simulink model "RL_Model_dyn"  (R2020a)
settings: Solver=FixedStepAuto  StartTime=0.0  StopTime=80  FixedStep=1E-3  MaxStep=0.01  MinStep=1e-3  RelTol=1e-3
model workspace (MAT data in the model file):
  reward_sys.DE_penalty_gain = 15
  reward_sys.DE_penalty_shape = 2
  reward_sys.HE_penalty_gain = 20
  reward_sys.HE_penalty_shape = 2
  reward_sys.HE_iwrt_DE = 1.5
  reward_sys.vel_reward_gain = 0
  reward_sys.vel_iwrt_DE = 1
  reward_sys.steering_penalty_gain = 0.1
  reward_sys.steering_iwrt_DE = 1
  reward_sys.steering_iwrt_HE = 1
values from neighbouring files (symbols this model uses):
  CP_Num = CP_Base_Num + CP_Wheels_Num    [init_Dmodel_sim_vars.m]
  D = 1000    [init_Dmodel_sim_vars.m]
  K = 1e6    (= 1000000)    [init_Dmodel_sim_vars.m]
  model = floatbase(model)    [init_Dmodel_sim_vars.m]
  Mu = 0.8    [init_Dmodel_sim_vars.m]
  q_init = [0 0 0 0]'    [init_Dmodel_sim_vars.m]
  qd_init = [0 0 0 0]'    [init_Dmodel_sim_vars.m]
  R = 0.1    [init_Dmodel_sim_vars.m]
  x_init = [1 0 0 0  0 0 zoff   0 0 0  2 0 0]'    [init_Dmodel_sim_vars.m]
undefined symbols (not defined in the file or in its folder): DiscIntNeverNeededParam, Fpt, gcontact, gcPosVel
libraries: simulink x7, rllib x1
settings Model: Creator=12248  LastModifiedBy=sky32
settings SolverCC: ZeroCrossAlgorithm=Adaptive
settings DataIOCC: SignalLogging=off
settings SFSimCC: CustomCodeUndefinedFunction=UseInterfaceOnly

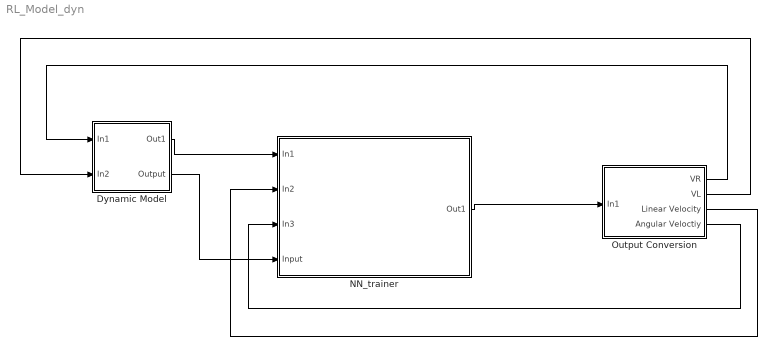
== system RL_Model_dyn ==
  Dynamic Model : Subsystem
  NN_trainer : Subsystem
  Output Conversion : Subsystem
  wires:
  NN_trainer/1(Out1) -> Output Conversion/1(In1)
  Dynamic Model/1(Out1) -> NN_trainer/1(In1)
  Output Conversion/4(Angular Veloctiy) -> NN_trainer/3(In3)
  Output Conversion/3(Linear Velocity) -> NN_trainer/2(In2)
  Output Conversion/1(VR) -> Dynamic Model/1(In1)
  Output Conversion/2(VL) -> Dynamic Model/2(In2)
  Dynamic Model/2(Output) -> NN_trainer/4(Input)

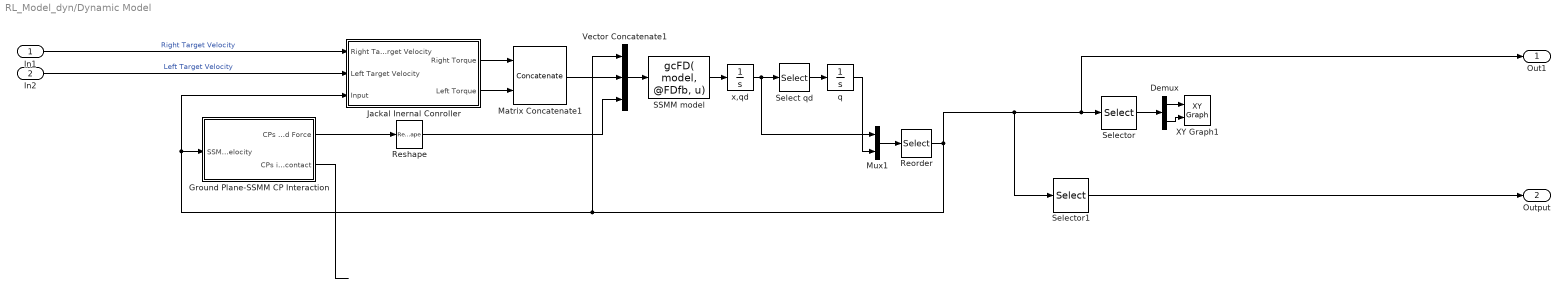
== system RL_Model_dyn/Dynamic Model ==
  In1 : Inport
  In2 : Inport  Port=2
  Demux : Demux  Outputs=2
  Ground Plane-SSMM CP Interaction : Subsystem
  Jackal Inernal Conroller : Subsystem
  Matrix Concatenate1 : Concatenate  Mode=Multidimensional array
  Mux1 : Mux  Inputs=2
  Reorder : Selector  InputPortWidth=21  IndexOptions=Index vector (dialog)  Indices=[1 2 3 4 5 6 7 8 9 10 11 12 13 18 19 20 21 14 15 16 17]  OutputSizes=1
  Reshape : Reshape  OutputDimensionality=Column vector (2-D)
  SSMM model : MATLABFcn  MATLABFcn=gcFD( model, @FDfb, u)  OutputDimensions=[17 1]  OutputSignalType=real  Output1D=off
  Select qd : Selector  InputPortWidth=17  IndexOptions=Index vector (dialog)  Indices=[14 15 16 17]  OutputSizes=1
  Selector : Selector  InputPortWidth=21  IndexOptions=Index vector (dialog)  Indices=[5 6]  OutputSizes=1
  Selector1 : Selector  InputPortWidth=21  IndexOptions=Index vector (dialog)  Indices=[10]  OutputSizes=1
  Vector Concatenate1 : Concatenate  NumInputs=3
  XY Graph1 : simulink/Sinks/XY Graph  xmin=graph_vars.x_lb  xmax=graph_vars.x_ub  ymin=graph_vars.y_lb  ymax=graph_vars.y_ub  st=-1
  q : Integrator  InitialCondition=q_init
  x,qd : Integrator  InitialCondition=[x_init;qd_init]
  Out1 : Outport  VectorParamsAs1DForOutWhenUnconnected=off
  Output : Outport  Port=2
  wires:
  Select qd/1 -> q/1
  Reorder/1 -> Vector Concatenate1/1, Ground Plane-SSMM CP Interaction/1(SSMM Position and Velocity), Jackal Inernal Conroller/3(Input), Selector1/1, Out1/1, Selector/1
  Demux/2 -> XY Graph1/2
  Selector/1 -> Demux/1
  SSMM model/1 -> x,qd/1
  Reshape/1 -> Vector Concatenate1/3
  x,qd/1 -> Select qd/1, Mux1/1
  Vector Concatenate1/1 -> SSMM model/1
  Mux1/1 -> Reorder/1
  Jackal Inernal Conroller/2(Left Torque) -> Matrix Concatenate1/2
  Demux/1 -> XY Graph1/1
  Ground Plane-SSMM CP Interaction/1(CPs Applied Force) -> Reshape/1
  q/1 -> Mux1/2
  Matrix Concatenate1/1 -> Vector Concatenate1/2
  Jackal Inernal Conroller/1(Right Torque) -> Matrix Concatenate1/1
  In1/1 -> Jackal Inernal Conroller/1(Right Target Velocity)  "Right Target Velocity"
  In2/1 -> Jackal Inernal Conroller/2(Left Target Velocity)  "Left Target Velocity"
  Ground Plane-SSMM CP Interaction/2(CPs in contact) -> ?
  Selector1/1 -> Output/1

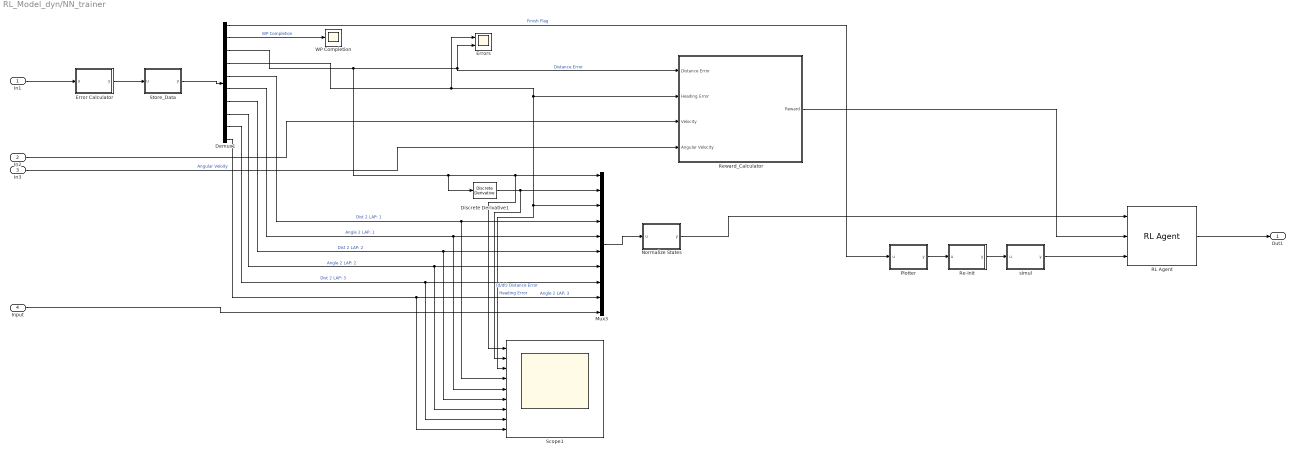
== system RL_Model_dyn/NN_trainer ==
  In1 : Inport
  In2 : Inport  Port=2
  In3 : Inport  Port=3
  Input : Inport  Port=4
  Demux1 : Demux  Outputs=10
  Discrete Derivative1 : simulink/Discrete/Discrete Derivative  gainval=1.0  ICPrevScaledInput=0.0  OutMin=[]  OutMax=[]  OutDataType=fixdt(1, 16)  OutScaling=2^-10  DoSatur=off
  Error Calculator : MATLAB Function  TreatAsAtomicUnit=on
  Errors : Scope  NumInputPorts=2
  Mux3 : Mux  Inputs=10
  Normalize States : MATLAB Function  TreatAsAtomicUnit=on
  Plotter : MATLAB Function  TreatAsAtomicUnit=on
  RL Agent : rllib/RL Agent  Agent=agent  ProvideReward=on  ProvideIsDone=on  ProvideCumRwd=off  TreatAsDirectFeedthrough=on  CollectLoggedSignals=on  CollectModelStates=on
  Re-Init : MATLAB Function  TreatAsAtomicUnit=on
  Reward_Calculator : Subsystem
  Scope1 : Scope  NumInputPorts=9
  Store_Data : MATLAB Function  TreatAsAtomicUnit=on
  WP Completion : Scope
  simul : MATLAB Function  TreatAsAtomicUnit=on
  Out1 : Outport  VectorParamsAs1DForOutWhenUnconnected=off
  wires:
  Re-Init/1(y) -> simul/1(u)
  Demux1/1 -> Plotter/1(u)  "Finish Flag"
  Plotter/1(y) -> Re-Init/1(u)
  In3/1 -> Reward_Calculator/4(Angular Velocity)  "Angular Veloity"
  In1/1 -> Error Calculator/1(u)
  RL Agent/1 -> Out1/1
  Demux1/2 -> WP Completion/1  "WP Completion"
  Store_Data/1(y) -> Demux1/1
  In2/1 -> Reward_Calculator/3(Velocity)
  Demux1/4 -> Scope1/3, Mux3/3, Reward_Calculator/2(Heading Error), Errors/1  "Heading Error"
  Normalize States/1(y) -> RL Agent/1
  Mux3/1 -> Normalize States/1(u)
  Discrete Derivative1/1 -> Scope1/2, Mux3/2  "(d/dt) Distance Error"
  Demux1/3 -> Errors/2, Reward_Calculator/1(Distance Error), Discrete Derivative1/1, Scope1/1, Mux3/1  "Distance Error"
  Reward_Calculator/1(Reward) -> RL Agent/2
  Demux1/5 -> Scope1/4, Mux3/4  "Dist 2 LAP: 1"
  Demux1/6 -> Scope1/5, Mux3/5  "Angle 2 LAP: 1"
  Demux1/7 -> Scope1/6, Mux3/6  "Dist 2 LAP: 2"
  Demux1/8 -> Scope1/7, Mux3/7  "Angle 2 LAP: 2"
  Demux1/9 -> Scope1/8, Mux3/8  "Dist 2 LAP: 3"
  Demux1/10 -> Scope1/9, Mux3/9  "Angle 2 LAP: 3"
  Input/1 -> Mux3/10
  Error Calculator/1(y) -> Store_Data/1(u)
  simul/1(y) -> RL Agent/3

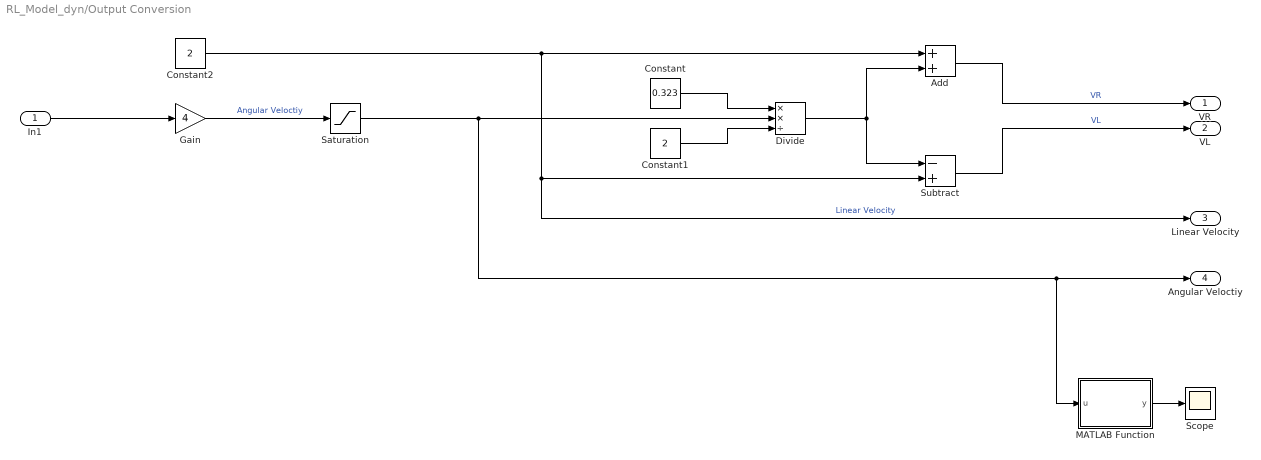
== system RL_Model_dyn/Output Conversion ==
  In1 : Inport
  Add : Sum
  Constant : Constant  Value=0.323
  Constant1 : Constant  Value=2
  Constant2 : Constant  Value=2
  Divide : Product  Inputs=**/
  Gain : Gain  Gain=4
  MATLAB Function : MATLAB Function  TreatAsAtomicUnit=on
  Saturation : Saturate  UpperLimit=4  LowerLimit=-4
  Scope : Scope
  Subtract : Sum  Inputs=-+
  VR : Outport  VectorParamsAs1DForOutWhenUnconnected=off
  VL : Outport  Port=2  VectorParamsAs1DForOutWhenUnconnected=off
  Linear Velocity : Outport  Port=3  VectorParamsAs1DForOutWhenUnconnected=off
  Angular Veloctiy : Outport  Port=4  VectorParamsAs1DForOutWhenUnconnected=off
  wires:
  In1/1 -> Gain/1
  Divide/1 -> Add/2, Subtract/1
  Constant2/1 -> Subtract/2, Linear Velocity/1, Add/1  "Linear Velocity"
  Constant1/1 -> Divide/3
  Gain/1 -> Saturation/1  "Angular Veloctiy"
  Subtract/1 -> VL/1  "VL"
  Constant/1 -> Divide/1
  Add/1 -> VR/1  "VR"
  MATLAB Function/1(y) -> Scope/1
  Saturation/1 -> Divide/2, Angular Veloctiy/1, MATLAB Function/1(u)

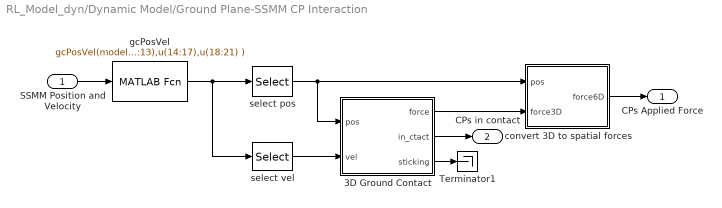
== system RL_Model_dyn/Dynamic Model/Ground Plane-SSMM CP Interaction ==
  SSMM Position and Velocity : Inport
  3D Ground Contact : Subsystem  mask(3D Nonlinear Ground Contact with Friction){K=K, D=D, mu=Mu, np=CP_Num}
      mask prompts: K "Stiffness (K)"; D "Damping (D)"; mu "Coefficient of Friction (mu)"; np "Number of Contact Points"
      mask help:
      | Given two 3xnp arrays containing contact-point positions and
      | velocities, calculate the 3xnp array of ground-reaction forces
      | acting on those points. Also calculate 1xnp boolean vectors
      | in_ctact (true if normal force >0) and sticking (true if inside
      | or on boundary of friction cone).  Zero-crossing detection is
      | enabled at both make/break contact and stick/slip transitions.
  Terminator1 : Terminator
  convert 3D to spatial forces : Subsystem
  gcPosVel : MATLABFcn  MATLABFcn=gcPosVel(model, u(1:13),u(14:17),u(18:21) )  OutputDimensions=[6 CP_Num]  OutputSignalType=real  Output1D=off
  select pos : Selector  NumberOfDimensions=2  InputPortWidth=3  IndexOptions=Index vector (dialog),Select all  Indices=[1 2 3],1  OutputSizes=1,1
  select vel : Selector  NumberOfDimensions=2  InputPortWidth=3  IndexOptions=Index vector (dialog),Select all  Indices=[4 5 6],1  OutputSizes=1,1
  CPs Applied Force : Outport  VectorParamsAs1DForOutWhenUnconnected=off
  CPs in contact : Outport  Port=2  VectorParamsAs1DForOutWhenUnconnected=off
  wires:
  gcPosVel/1 -> select vel/1, select pos/1
  select pos/1 -> convert 3D to spatial forces/1(pos), 3D Ground Contact/1(pos)
  convert 3D to spatial forces/1(force6D) -> CPs Applied Force/1
  select vel/1 -> 3D Ground Contact/2(vel)
  3D Ground Contact/3(sticking) -> Terminator1/1
  3D Ground Contact/2(in_ctact) -> CPs in contact/1
  SSMM Position and Velocity/1 -> gcPosVel/1
  3D Ground Contact/1(force) -> convert 3D to spatial forces/2(force3D)

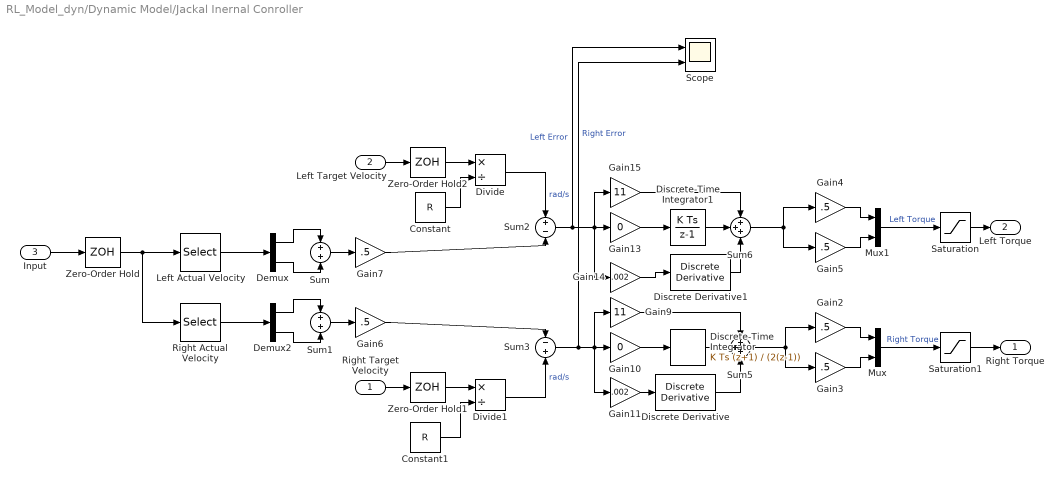
== system RL_Model_dyn/Dynamic Model/Jackal Inernal Conroller ==
  Right Target Velocity : Inport
  Left Target Velocity : Inport  Port=2
  Input : Inport  Port=3
  Constant : Constant  Value=R
  Constant1 : Constant  Value=R
  Demux : Demux  Outputs=2
  Demux2 : Demux  Outputs=2
  Discrete Derivative : simulink/Discrete/Discrete Derivative  gainval=1  ICPrevScaledInput=0.0  OutMin=[]  OutMax=[]  OutDataType=fixdt(1, 16)  OutScaling=2^-10  DoSatur=off
  Discrete Derivative1 : simulink/Discrete/Discrete Derivative  gainval=1  ICPrevScaledInput=0.0  OutMin=[]  OutMax=[]  OutDataType=fixdt(1, 16)  OutScaling=2^-10  DoSatur=off
  Discrete-Time Integrator : DiscreteIntegrator  IntegratorMethod=Integration: Trapezoidal  SampleTime=-1  ICPrevOutput=DiscIntNeverNeededParam  ICPrevScaledInput=DiscIntNeverNeededParam
  Discrete-Time Integrator1 : DiscreteIntegrator  SampleTime=-1  ICPrevOutput=DiscIntNeverNeededParam  ICPrevScaledInput=DiscIntNeverNeededParam
  Divide : Product  Inputs=*/
  Divide1 : Product  Inputs=*/
  Gain10 : Gain  Gain=0
  Gain11 : Gain  Gain=.002
  Gain13 : Gain  Gain=0
  Gain14 : Gain  Gain=.002
  Gain15 : Gain  Gain=11
  Gain{2..7} (6 alike) : Gain  Gain=.5
  Gain9 : Gain  Gain=11
  Left Actual Velocity : Selector  InputPortWidth=21  IndexOptions=Index vector (dialog)  Indices=[20 21]  OutputSizes=1
  Mux : Mux  Inputs=2
  Mux1 : Mux  Inputs=2
  Right Actual Velocity : Selector  InputPortWidth=21  IndexOptions=Index vector (dialog)  Indices=[18 19]  OutputSizes=1
  Saturation : Saturate  UpperLimit=1000  LowerLimit=-1000
  Saturation1 : Saturate  UpperLimit=1000  LowerLimit=-1000
  Scope : Scope  NumInputPorts=2
  Sum : Sum  Inputs=2
  Sum1 : Sum  Inputs=2
  Sum2 : Sum  Inputs=+-
  Sum3 : Sum  Inputs=-+
  Sum5 : Sum  Inputs=+++
  Sum6 : Sum  Inputs=+++
  Zero-Order Hold : ZeroOrderHold  SampleTime=.001
  Zero-Order Hold1 : ZeroOrderHold  SampleTime=.001
  Zero-Order Hold2 : ZeroOrderHold  SampleTime=.001
  Right Torque : Outport  VectorParamsAs1DForOutWhenUnconnected=off
  Left Torque : Outport  Port=2  VectorParamsAs1DForOutWhenUnconnected=off
  wires:
  Gain3/1 -> Mux/2
  Input/1 -> Zero-Order Hold/1
  Left Actual Velocity/1 -> Demux/1
  Demux/1 -> Sum/1
  Demux/2 -> Sum/2
  Demux2/1 -> Sum1/1
  Demux2/2 -> Sum1/2
  Right Actual Velocity/1 -> Demux2/1
  Sum1/1 -> Gain6/1
  Sum/1 -> Gain7/1
  Gain6/1 -> Sum3/1
  Sum3/1 -> Scope/2, Gain9/1, Gain11/1, Gain10/1  "Right Error"
  Gain9/1 -> Sum5/1
  Gain10/1 -> Discrete-Time Integrator/1
  Gain4/1 -> Mux1/1
  Gain5/1 -> Mux1/2
  Left Target Velocity/1 -> Zero-Order Hold2/1
  Constant/1 -> Divide/2
  Divide/1 -> Sum2/1  "rad/s"
  Constant1/1 -> Divide1/2
  Divide1/1 -> Sum3/2  "rad/s"
  Gain7/1 -> Sum2/2
  Gain2/1 -> Mux/1
  Mux1/1 -> Saturation/1  "Left Torque"
  Mux/1 -> Saturation1/1  "Right Torque"
  Sum5/1 -> Gain3/1, Gain2/1
  Zero-Order Hold/1 -> Right Actual Velocity/1, Left Actual Velocity/1
  Right Target Velocity/1 -> Zero-Order Hold1/1
  Zero-Order Hold1/1 -> Divide1/1
  Zero-Order Hold2/1 -> Divide/1
  Gain11/1 -> Discrete Derivative/1
  Discrete Derivative/1 -> Sum5/3
  Discrete-Time Integrator/1 -> Sum5/2
  Gain14/1 -> Discrete Derivative1/1
  Gain13/1 -> Discrete-Time Integrator1/1
  Sum2/1 -> Scope/1, Gain15/1, Gain14/1, Gain13/1  "Left Error"
  Discrete Derivative1/1 -> Sum6/3
  Sum6/1 -> Gain5/1, Gain4/1
  Gain15/1 -> Sum6/1
  Discrete-Time Integrator1/1 -> Sum6/2
  Saturation/1 -> Left Torque/1
  Saturation1/1 -> Right Torque/1

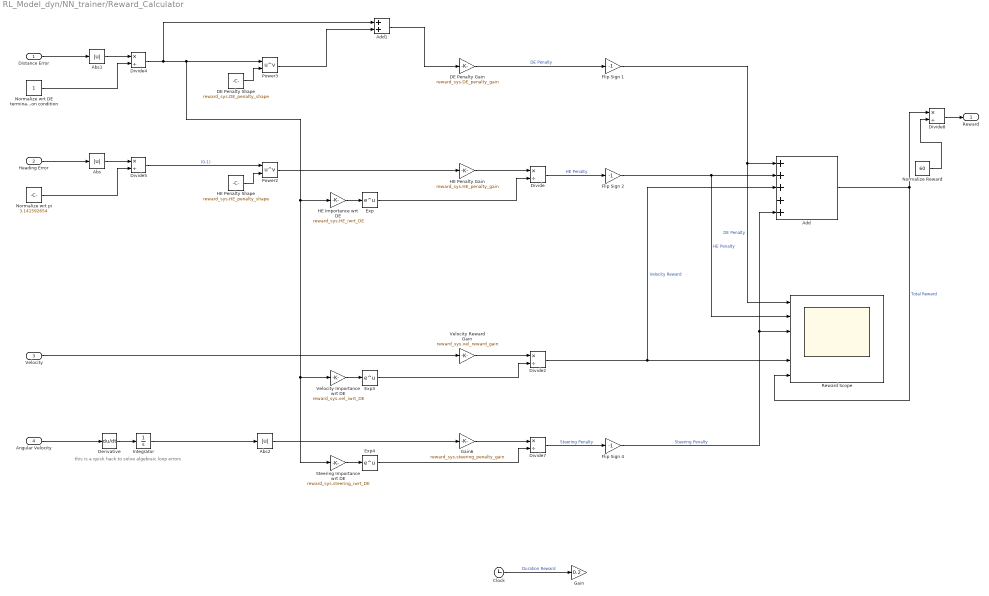
== system RL_Model_dyn/NN_trainer/Reward_Calculator ==
  note: this is a quick hack to solve algebraic loop errors
  Distance Error : Inport
  Heading Error : Inport  Port=2
  Velocity : Inport  Port=3
  Angular Velocity : Inport  Port=4
  Abs : Abs
  Abs1 : Abs
  Abs2 : Abs
  Add : Sum  Inputs=+++++
  Add1 : Sum
  Clock : Clock
  DE Penalty Gain : Gain  Gain=reward_sys.DE_penalty_gain
  DE Penalty Shape : Constant  Value=reward_sys.DE_penalty_shape
  Derivative : Derivative
  Divide{,2,4..5,7..8} (6 alike) : Product  Inputs=*/
  Exp : Math  SignedPower=on  SaturateOnIntegerOverflow=on
  Exp3 : Math  SignedPower=on  SaturateOnIntegerOverflow=on
  Exp4 : Math  SignedPower=on  SaturateOnIntegerOverflow=on
  Flip Sign 1 : Gain  Gain=-1
  "Flip Sign 2 " : Gain  Gain=-1
  Flip Sign 4 : Gain  Gain=-1
  Gain : Gain  Gain=0.2
  Gain6 : Gain  Gain=reward_sys.steering_penalty_gain
  HE Importance wrt DE : Gain  Gain=reward_sys.HE_iwrt_DE
  HE Penalty Gain : Gain  Gain=reward_sys.HE_penalty_gain
  HE Penalty Shape : Constant  Value=reward_sys.HE_penalty_shape
  Integrator : Integrator
  Normalize Reward : Constant  Value=60
  Normalize wrt DE termination condition : Constant
  Normalize wrt pi : Constant  Value=3.141592654
  Power2 : Math  Operator=pow  SignedPower=on  SaturateOnIntegerOverflow=on
  Power3 : Math  Operator=pow  SignedPower=on  SaturateOnIntegerOverflow=on
  Reward Scope : Scope  NumInputPorts=6
  Steering Importance wrt DE : Gain  Gain=reward_sys.steering_iwrt_DE
  Velocity Importance wrt DE : Gain  Gain=reward_sys.vel_iwrt_DE
  Velocity Reward Gain : Gain  Gain=reward_sys.vel_reward_gain
  Reward : Outport  VectorParamsAs1DForOutWhenUnconnected=off
  wires:
  Heading Error/1 -> Abs/1
  Distance Error/1 -> Abs1/1
  Add/1 -> Reward Scope/6, Divide8/1  "Total Reward"
  Divide/1 -> "Flip Sign 2 "/1  "HE Penalty"
  DE Penalty Gain/1 -> Flip Sign 1/1  "DE Penalty"
  Divide4/1 -> Add1/1, Power3/1, Steering Importance wrt DE/1, Velocity Importance wrt DE/1, HE Importance wrt DE/1
  Velocity/1 -> Velocity Reward Gain/1
  Divide2/1 -> Add/3, Reward Scope/5  "Velocity Reward"
  HE Importance wrt DE/1 -> Exp/1
  HE Penalty Gain/1 -> Divide/1
  Exp/1 -> Divide/2
  Velocity Reward Gain/1 -> Divide2/1
  Velocity Importance wrt DE/1 -> Exp3/1
  Exp3/1 -> Divide2/2
  Abs1/1 -> Divide4/1
  Normalize wrt DE termination condition/1 -> Divide4/2
  Abs/1 -> Divide5/1
  Normalize wrt pi/1 -> Divide5/2
  Divide5/1 -> Power2/1  "(0-1)"
  Power2/1 -> HE Penalty Gain/1
  HE Penalty Shape/1 -> Power2/2
  DE Penalty Shape/1 -> Power3/2
  Angular Velocity/1 -> Derivative/1
  Gain6/1 -> Divide7/1
  Steering Importance wrt DE/1 -> Exp4/1
  Exp4/1 -> Divide7/2
  Divide7/1 -> Flip Sign 4/1  "Steering Penalty"
  Abs2/1 -> Gain6/1
  Divide8/1 -> Reward/1
  Normalize Reward/1 -> Divide8/2
  Flip Sign 1/1 -> Add/1, Reward Scope/1  "DE Penalty"
  "Flip Sign 2 "/1 -> Reward Scope/2, Add/2  "HE Penalty"
  Flip Sign 4/1 -> Add/5, Reward Scope/3  "Steering Penalty"
  Clock/1 -> Gain/1  "Duration Reward"
  Power3/1 -> Add1/2
  Add1/1 -> DE Penalty Gain/1
  Derivative/1 -> Integrator/1
  Integrator/1 -> Abs2/1

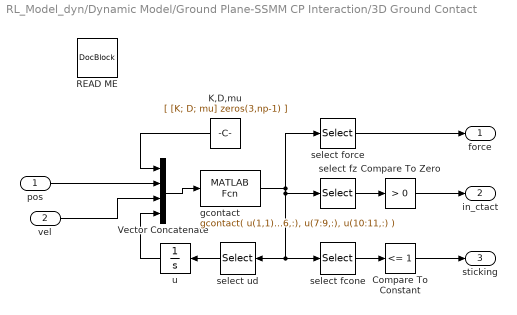
== system RL_Model_dyn/Dynamic Model/Ground Plane-SSMM CP Interaction/3D Ground Contact ==
  pos : Inport
  vel : Inport  Port=2
  Compare To Constant : simulink/Logic and Bit Operations/Compare To Constant  relop=<=  const=1  OutDataTypeStr=boolean
  Compare To Zero : simulink/Logic and Bit Operations/Compare To Zero  relop=>  OutDataTypeStr=boolean
  K,D,mu : Constant  Value=[ [K; D; mu] zeros(3,np-1) ]  VectorParams1D=off
  READ ME : simulink/Model-Wide Utilities/DocBlock  DocumentType=Text
      content=|
      | The constant block supplies the parameters K, D and mu to the function
      | gcontact.  This is necessary because K, D and mu are defined in the
      | workspace of this particular masked subsystem, but the executable
      | expression in the "MATLAB Function" block does not have access to this
      | workspace, so the symbols K, D and mu cannot appear directly in the
      | executable expression.
      |
      | The ">0" block and the "<=1" block both have zero-crossing enabled.  The
      | former detects transitions between contact and non-contact, whereas the
      | latter detects transitions between sticking (due to friction) and
      | slipping.  A point can be sticking only if it is also in contact.  A
      | zero-crossing event occurs whenever any one point makes a transition.
      |
      | The state variable, u, is a 2x(np) matrix containing the horizontal
      | component of the local ground deformation for each point.  This quantity
      | is used to calculate the tangential (i.e., frictional) component of the
      | ground reaction force.
      |
      | When a point loses contact, its associated state variable, u(:,i), decays
      | to zero with a time constant of D/K.  If this ratio is small then the
      | corresponding differential equation is fast, and it is necessary to use
      | small integration time steps.  For example, if K=1e6 and D=2000 then
      | D/K=0.002 and u(:,i) decays in proportion to exp(-500t).  Increasing K
      | makes the surface stiffer, and decreasing D/K makes it bouncier, but the
      | latter also makes the post-contact recovery faster.  The degree of
      | bounciness depends on the mass of the impacting body: a heavier body will
      | bounce more.
      |
      | To adapt this subsystem to work in 2D, the only things that change are the
      | row dimensions of various matrices.  You will have to alter the row
      | selections in the executable expression in the "MATLAB Function" block,
      | and also the dimensions of its output matrix, and you will have to change
      | the row selections in the various "select" blocks.
      |
      | For more information, see "The Simulink Ground Contact Model" in the
      | spatial_v2 documentation directory.
  Vector Concatenate : Concatenate  NumInputs=4  Mode=Multidimensional array
  gcontact : MATLABFcn  MATLABFcn=gcontact( u(1,1), u(2,1), u(3,1), u(4:6,:), u(7:9,:), u(10:11,:) )  OutputDimensions=[6 np]  OutputSignalType=real  Output1D=off
  select fcone : Selector  NumberOfDimensions=2  InputPortWidth=3  IndexOptions=Index vector (dialog),Select all  Indices=[6],1  OutputSizes=1,1
  select force : Selector  NumberOfDimensions=2  InputPortWidth=3  IndexOptions=Index vector (dialog),Select all  Indices=[1 2 3],1  OutputSizes=1,1
  select fz : Selector  NumberOfDimensions=2  InputPortWidth=3  IndexOptions=Index vector (dialog),Select all  Indices=[3],1  OutputSizes=1,1
  select ud : Selector  NumberOfDimensions=2  InputPortWidth=3  IndexOptions=Index vector (dialog),Select all  Indices=[4 5],1  OutputSizes=1,1
  u : Integrator
  force : Outport  VectorParamsAs1DForOutWhenUnconnected=off
  in_ctact : Outport  Port=2  VectorParamsAs1DForOutWhenUnconnected=off
  sticking : Outport  Port=3  VectorParamsAs1DForOutWhenUnconnected=off
  wires:
  Vector Concatenate/1 -> gcontact/1
  select ud/1 -> u/1
  gcontact/1 -> select fz/1, select ud/1, select fcone/1, select force/1
  select fz/1 -> Compare To Zero/1
  select fcone/1 -> Compare To Constant/1
  Compare To Constant/1 -> sticking/1
  u/1 -> Vector Concatenate/4
  pos/1 -> Vector Concatenate/2
  K,D,mu/1 -> Vector Concatenate/1
  vel/1 -> Vector Concatenate/3
  Compare To Zero/1 -> in_ctact/1
  select force/1 -> force/1

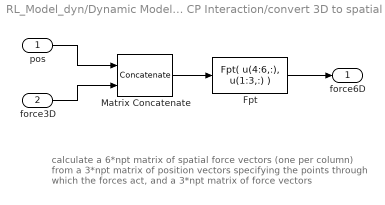
== system RL_Model_dyn/Dynamic Model/Ground Plane-SSMM CP Interaction/convert 3D to spatial forces ==
  note: calculate a 6*npt matrix of spatial force vectors (one per column)
      | from a 3*npt matrix of position vectors specifying the points
      | through which the forces act, and a 3*npt matrix of force vectors
  pos : Inport
  force3D : Inport  Port=2
  Fpt : MATLABFcn  MATLABFcn=Fpt( u(4:6,:), u(1:3,:) )  OutputSignalType=real  Output1D=off
  Matrix Concatenate : Concatenate  Mode=Multidimensional array
  force6D : Outport  VectorParamsAs1DForOutWhenUnconnected=off
  wires:
  force3D/1 -> Matrix Concatenate/2
  pos/1 -> Matrix Concatenate/1
  Matrix Concatenate/1 -> Fpt/1
  Fpt/1 -> force6D/1

== matlab function RL_Model_dyn/NN_trainer/Re-Init ==
  data: u input; y output
function y = fcn(u)

coder.extrinsic('assignin', 'evalin', 'trainRand', 'gen_graph_vars');

persistent termFlag;
if isempty(termFlag)
    termFlag = true;
end

if (u && termFlag)
    
    % set WPidx to 1 and assign to workspace
    WPidx = 1;
    assignin('base', 'WPidx', WPidx);
    
%     disp('re-init')
    %trainRand;
    gen_graph_vars;
    
    termFlag = false;
    
end
    
y = u;

== matlab function RL_Model_dyn/NN_trainer/Store_Data ==
  settings: updateMethod=DISCRETE  sampleTime=1e-2
  data: u input; y output
function y = fcn(u)

coder.extrinsic('evalin', 'assignin');


ang_velocity = 0;
ang_velocity = evalin('base', 'ang_velocity');

% flag that is true if it is the first time step of the simulation
persistent firstFlag;
if isempty(firstFlag)
    firstFlag = true;
end

if firstFlag
    % initialize temp_position_data array, this stores x-y coords
    % inintialize temp_error_data array, this stores distance error
    temp_position_data = [u(1), u(2)];
    temp_error_data = [u(5)];
    assignin('base', 'temp_position_data', temp_position_data);
    assignin('base', 'temp_error_data', temp_error_data);
    
    temp_error_for_nn_emul = [ang_velocity u(5) u(6) u(8) u(10) u(12)];
    assignin('base', 'temp_error_for_nn_emul', temp_error_for_nn_emul);
    
    firstFlag = false;
else
    temp_position_data = evalin('base', 'temp_position_data');
    temp_position_data = [temp_position_data;
                          u(1), u(2)];
    temp_error_data = evalin('base', 'temp_error_data');
    temp_error_data = [temp_error_data;
                       u(5)];
    assignin('base', 'temp_position_data', temp_position_data);
    assignin('base', 'temp_error_data', temp_error_data);
    
    %error for NN emulator
    temp_error_for_nn_emul = evalin('base', 'temp_error_for_nn_emul');
    temp_error_for_nn_emul = [temp_error_for_nn_emul;
                              ang_velocity u(5) u(6) u(8) u(10) u(12)];
    assignin('base', 'temp_error_for_nn_emul', temp_error_for_nn_emul);
end

y = u(3:12);

== matlab function RL_Model_dyn/NN_trainer/Normalize States ==
  data: u input; y output
function y = fcn(u)

%linVel = u(1);

PE = u(1);
dPE = u(2);
HE = u(3);
%TD = u(4);
%TA = u(5);
dist2LAP_1 = u(4);
rAng2LAP_1 = u(5);
dist2LAP_2 = u(6);
rAng2LAP_2 = u(7);
dist2LAP_3 = u(8);
rAng2LAP_3 = u(9);
angVel = u(10);

%linVel = linVel / 2;
%angVel = angVel / 3;

dPE = dPE / 2;
HE = HE / pi;
%TD = TD / 10;
%TA = TA / pi;
dist2LAP_1 = dist2LAP_1 / 2;
rAng2LAP_1 = rAng2LAP_1 / pi;
dist2LAP_2 = dist2LAP_2 / 3;
rAng2LAP_2 = rAng2LAP_2 / pi;
dist2LAP_3 = dist2LAP_3 / 4;
rAng2LAP_3 = rAng2LAP_3 / pi;
angVel = angVel / 4;


y = [PE;
     dPE;
     HE;
     dist2LAP_1;
     rAng2LAP_1;
     dist2LAP_2;
     rAng2LAP_2;
     dist2LAP_3;
     rAng2LAP_3;
     angVel];

== matlab function RL_Model_dyn/NN_trainer/Error Calculator ==
  settings: updateMethod=DISCRETE  sampleTime=1e-2
  data: u input; y output

% calculates distance error (the perpendicular distance from the robot's
% current position to a straight line between the previous waypoint and the
% target waypoint) and heading error, to be used as inputs to train a neural
% net

function y = fcn(u)
coder.extrinsic('evalin', 'assignin'); % seems like this might be important for avoiding errors during autocode generation (see how the pure pursuit code was structured in 8-1 deliverable if any issues occurr)

% (maybe make these persistent variables as well to increase runtime
% efficiency)
% Set class of numWP and read in from workspace
numWP = 0;
numWP = evalin('base', 'numWP');
% Set class of waypoints and read in from workspace
waypoints = zeros(numWP, 2);
waypoints = evalin('base', 'waypoints');
% Set class of WPidx and read in from workspace
WPidx = 0;
WPidx = evalin('base', 'WPidx');

% Initialize finish flag, waypoint index, and current path trajectory as persistent variables
% Finish flag
persistent finishFlag;
if isempty(finishFlag)
    finishFlag = false;
end

% Current path trajectory
persistent gAngCurrPath;
if isempty(gAngCurrPath)
    origin = [0, 0];
    wp1 = waypoints(1, :);
    gAngCurrPath = computeGlobalAngle(origin, wp1);
end

% Initialize distErr, headingErr, targDist, turnAng, dist2LAP, and rAng2LAP
% as persistent variables
persistent distErr;
if isempty(distErr)
    distErr = 0;
end
persistent headingErr;
if isempty(headingErr)
    headingErr = 0;
end
persistent dist2LAP_1;
if isempty(dist2LAP_1)
    dist2LAP_1 = 0;
end
persistent rAng2LAP_1;
if isempty(rAng2LAP_1)
    rAng2LAP_1 = 0;
end
persistent dist2LAP_2;
if isempty(dist2LAP_2)
    dist2LAP_2 = 0;
end
persistent rAng2LAP_2;
if isempty(rAng2LAP_2)
    rAng2LAP_2 = 0;
end
persistent dist2LAP_3;
if isempty(dist2LAP_3)
    dist2LAP_3 = 0;
end
persistent rAng2LAP_3;
if isempty(rAng2LAP_3)
    rAng2LAP_3 = 0;
end

% Initialize waypoint completion flag
WPcompletion = false;

%######################################################################
%======================================================================

% COMMENT/UNCOMMENT DEPENDING ON MODEL BEING USED

%========================== DYNAMIC MODEL =============================
% extract current robot position [x, y]
currPos = [u(5), u(6)];
% extract orientation quaternion
q = [u(1), u(2), u(3), u(4)];
% compute angle robot is currently facing
currAng = atan2(2 * (q(1) * q(4) + q(2) * q(3)), 1 - 2 * (q(3)^2 + q(4)^2));
%========================== KINEMATIC MODEL ===========================
% % extract current robot position [x, y]
% currPos = [u(1), u(2)];
% % extract current angle
% currAng = u(3);
%======================================================================
%######################################################################
% disp('finishFlag:')
% disp(finishFlag)
% if the simulation has finished (this is to deal with Simulink termination
% condition unexpected behavior)
if (finishFlag == true)
    
    y = [currPos(1), currPos(2), finishFlag, WPcompletion, distErr, headingErr, dist2LAP_1, rAng2LAP_1, dist2LAP_2, rAng2LAP_2, dist2LAP_3, rAng2LAP_3];
    
% else the simulation is not finished
else
    
    % set target waypoint
    targWP = waypoints(WPidx, :);
    % compute distance to target waypoint
    targDist = pythag(currPos, targWP);
    % compute turn angle
    turnAng = computeTurnAngle(WPidx, numWP, waypoints);
    % if robot still has yet to reach 1st waypoint
    if(WPidx == 1)
        % set previous waypoint to the origin
        % *** NOT VALID IF ROBOT IS INITIALIZED ELSEWHERE THAN THE ORIGIN ***
        prevWP = [0, 0];
    else
        % set previous waypoint
        prevWP = waypoints(WPidx-1, :);
    end
    
    
    
    lookAheadPt = lookAheadPoint(3, waypoints, numWP, WPidx, prevWP, targWP, currPos);
    dist2LAP = pythag(currPos, lookAheadPt);
    gAng2LAP = computeGlobalAngle(currPos, lookAheadPt);
    rAng2LAP = computeRelativeAngle(currAng, gAng2LAP);
    
    
    
    % compute the global angle of current position wrt target waypoint
    gAngCPwrtTarg = computeGlobalAngle(targWP, currPos);
    
    %######################################################################
    %======================================================================
    % THIS DETERMINES WAYPOINT COMPLETION CRITERIA, ONLY ONE OF THESE IS TO
    % BE USED IN THE WHILE LOOP BELOW
    %======================================================================
    % compute the relative angle between the (current position wrt target waypoint) and the (current path trajectory)
    rAngCPwrtTarg = computeRelativeAngle(gAngCurrPath, gAngCPwrtTarg);
    %======================================================================
    % compute global bisector angle
    gBiAng = computeBiAng(gAngCurrPath, turnAng);
    % compute relative angle between (current position wrt target WP) and (bisector angle)
    rAngCPwrtBi = computeRelativeAngle(gBiAng, gAngCPwrtTarg);
    %======================================================================
    %######################################################################
    
%     disp('-----------------')
%     disp(['currPos = (', sprintf('%5.2f', currPos(1)), ', ', sprintf('%5.2f', currPos(2)), ')']);
%     disp(['targWP = (', sprintf('%5.2f', targWP(1)), ', ', sprintf('%5.2f', targWP(2)), ')']);
%     disp(['gAngCPwrtTarg = ', sprintf('%5.2f', gAngCPwrtTarg)]);
%     disp(['gBiAng = ', sprintf('%5.2f', gBiAng)]);
%     disp(['rAngCPwrtBi = ', sprintf('%5.2f', rAngCPwrtBi), ' <= ', sprintf('%5.2f', pi/2)]);
%     disp('-----------------')
    
    % while the robot has crossed the line defining the waypoint completion
    % criteria (it is more intuitive to think of this as an if condition,
    % but a while loop is used to deal with the edge case where the robot
    % passes 2 waypoints in a single timestep)
    while (abs(rAngCPwrtBi) <= (pi / 2))
%         disp('WP completed');
        % set waypoint completion
        WPcompletion = true;
        % increment WPidx and assign to base workspace
        WPidx = WPidx + 1;
        assignin('base', 'WPidx', WPidx);
        % if the last waypoint has been reached
        if(WPidx > numWP)
            % set finiishflag to true
            finishFlag = true;

            y = [currPos(1), currPos(2), finishFlag, WPcompletion, distErr, headingErr, dist2LAP_1, rAng2LAP_1, dist2LAP_2, rAng2LAP_2, dist2LAP_3, rAng2LAP_3];
            
            % when this point is reached, the simulation has finished
            return
        % else there is another waypoint
        else
            % set previous waypoint
            prevWP = targWP;
            % set coordinates of the new target waypoint
            targWP = waypoints(WPidx, :);
            % compute distance to new target waypoint
            targDist = pythag(currPos, targWP);
            % compute turn angle
            turnAng = computeTurnAngle(WPidx, numWP, waypoints);
            % compute the new current path trajectory and write to workspace
            gAngCurrPath = computeGlobalAngle(prevWP, targWP);
            % compute the new angle of current position wrt target waypoint
            gAngCPwrtTarg = computeGlobalAngle(targWP, currPos);
            
            % compute the new relative angle between the (current position wrt target waypoint) and the (current path trajectory)
            rAngCPwrtTarg = computeRelativeAngle(gAngCurrPath, gAngCPwrtTarg);
            % compute the new global bisector angle
            gBiAng = computeBiAng(gAngCurrPath, turnAng);
            % compute the new relative angle between (current position wrt target WP) and (bisector angle)
            rAngCPwrtBi = computeRelativeAngle(gBiAng, gAngCPwrtTarg);
            
            % Compute Look Ahead Point 1
            lookAheadPt_1 = lookAheadPoint(1, waypoints, numWP, WPidx, prevWP, targWP, currPos);
            dist2LAP_1 = pythag(currPos, lookAheadPt_1);
            gAng2LAP_1 = computeGlobalAngle(currPos, lookAheadPt_1);
            rAng2LAP_1 = computeRelativeAngle(currAng, gAng2LAP_1);
            
            % Compute Look Ahead Point 2
            lookAheadPt_2 = lookAheadPoint(2, waypoints, numWP, WPidx, prevWP, targWP, currPos);
            dist2LAP_2 = pythag(currPos, lookAheadPt_2);
            gAng2LAP_2 = computeGlobalAngle(currPos, lookAheadPt_2);
            rAng2LAP_2 = computeRelativeAngle(currAng, gAng2LAP_2);
            
            % Compute Look Ahead Point 3
            lookAheadPt_3 = lookAheadPoint(3, waypoints, numWP, WPidx, prevWP, targWP, currPos);
            dist2LAP_3 = pythag(currPos, lookAheadPt_3);
            gAng2LAP_3 = computeGlobalAngle(currPos, lookAheadPt_3);
            rAng2LAP_3 = computeRelativeAngle(currAng, gAng2LAP_3);
            
        end
    end
    
    % compute path heading error
    headingErr = computeRelativeAngle(gAngCurrPath, currAng);
    % compute distance error
    distErr = distanceError(currPos, prevWP, targWP);
    % set sign (+/-) of distance error
    if (rAngCPwrtTarg < 0)
        distErr = -distErr;
    end
    
    if (abs(distErr) > 1)
        finishFlag = true;
    end

    % Compute Look Ahead Point 1
    lookAheadPt_1 = lookAheadPoint(1, waypoints, numWP, WPidx, prevWP, targWP, currPos);
    dist2LAP_1 = pythag(currPos, lookAheadPt_1);
    gAng2LAP_1 = computeGlobalAngle(currPos, lookAheadPt_1);
    rAng2LAP_1 = computeRelativeAngle(currAng, gAng2LAP_1);

    % Compute Look Ahead Point 2
    lookAheadPt_2 = lookAheadPoint(2, waypoints, numWP, WPidx, prevWP, targWP, currPos);
    dist2LAP_2 = pythag(currPos, lookAheadPt_2);
    gAng2LAP_2 = computeGlobalAngle(currPos, lookAheadPt_2);
    rAng2LAP_2 = computeRelativeAngle(currAng, gAng2LAP_2);

    % Compute Look Ahead Point 3
    lookAheadPt_3 = lookAheadPoint(3, waypoints, numWP, WPidx, prevWP, targWP, currPos);
    dist2LAP_3 = pythag(currPos, lookAheadPt_3);
    gAng2LAP_3 = computeGlobalAngle(currPos, lookAheadPt_3);
    rAng2LAP_3 = computeRelativeAngle(currAng, gAng2LAP_3);
    
    % Set return values
    y = [currPos(1), currPos(2), finishFlag, WPcompletion, distErr, headingErr, dist2LAP_1, rAng2LAP_1, dist2LAP_2, rAng2LAP_2, dist2LAP_3, rAng2LAP_3];

end

end


%========================= HELPER FUNCTIONS ===============================

function ret = lookAheadPoint(lookAheadDist, waypoints, numWP, WPidx, prevWP, targWP, currPos)

dist2go = lookAheadDist;
%!! make sure this doesn't deepcopy WPidx
refIdx = WPidx;

nP = nearestPoint(prevWP, targWP, currPos);

% distance down the path to the next waypoint
nextDist = pythag(nP, targWP);
% while the look-ahead point is not on the current path segment
while (nextDist < dist2go)
    if (refIdx == numWP)
        break;
    end
    dist2go = dist2go - nextDist;
    refIdx = refIdx + 1;
    prevWP = waypoints(refIdx-1, :);
    targWP = waypoints(refIdx, :);
    nextDist = pythag(prevWP, targWP);
end

x_component = (targWP(1) - prevWP(1)) / pythag(prevWP, targWP);
y_component = (targWP(2) - prevWP(2)) / pythag(prevWP, targWP);

if (refIdx == WPidx)
    x_LAP = currPos(1) + dist2go * x_component;
    y_LAP = currPos(2) + dist2go * y_component;
else
    x_LAP = prevWP(1) + dist2go * x_component;
    y_LAP = prevWP(2) + dist2go * y_component;
end

ret = [x_LAP, y_LAP];

end

% compute nearest point on the current path segment
function ret = nearestPoint(prevWP, targWP, currPos)
% compute equation of current path segment of form ax + by + c = 0
a = (prevWP(2) - targWP(2)) / (targWP(1) - prevWP(1));
b = 1;
c = ((targWP(2) - prevWP(2)) / (targWP(1) - prevWP(1))) * prevWP(1) - prevWP(2);

x_ret = (b * (b * currPos(1) - a * currPos(2)) - a * c) / (a * a + b * b);
y_ret = (a * (-b * currPos(1) + a * currPos(2)) - b * c) / (a * a + b * b);

ret = [x_ret, y_ret];
end

% compute bisector angle
function ret = computeBiAng(gAngCurrPath, turnAng)

ret = gAngCurrPath + (turnAng / 2);

ret = abs_lt_pi(ret);

end

% compute turn angle
function ret = computeTurnAngle(WPidx, numWP, waypoints)
% if a waypoint exists beyond the target waypoint
if (WPidx < numWP)
    % if robot still has yet to reach 1st waypoint
    if(WPidx == 1)
        % set previous waypoint to the origin
        % *** NOT VALID IF ROBOT IS INITIALIZED ELSEWHERE THAN THE ORIGIN ***
        prevWP = [0, 0];
    else
        % set previous waypoint
        prevWP = waypoints(WPidx-1, :);
    end
    % set target waypoint
    targWP = waypoints(WPidx, :);
    % set next target waypoint
    nextTarg = waypoints(WPidx+1, :);
    % compute global angle of target waypoint wrt previous waypoint
    % (aka the global angle of the current trajectory)
    angCT_glob = computeGlobalAngle(prevWP, targWP);
    % compute global angle of next target waypoint wrt target waypoint
    % (aka the global angle of the next trajectory)
    angNT_glob = computeGlobalAngle(targWP, nextTarg);
    % compute relative angle of next trajectory wrt current trajectory
    ret = computeRelativeAngle(angCT_glob, angNT_glob);
else
    ret = 0;
end

end


% pythagorean theorem
function h = pythag(p1, p2)

h = sqrt((p1(1) - p2(1))^2 + (p1(2) - p2(2))^2);

end


% input:  coordinate pairs describing positions of current robot position,
%         previous waypoint position, and target waypoint position
% output: perpendicular distance between current robot position and a
%         straight line connecting previous waypoint to target waypoint

function distErr = distanceError(currPos, prevWP, targWP)

x0 = currPos(1);
y0 = currPos(2);
x1 = prevWP(1);
y1 = prevWP(2);
x2 = targWP(1);
y2 = targWP(2);

distErr = abs(x0 * (y2 - y1) - y0 * (x2 - x1) + x2 * y1 - y2 * x1) / sqrt((y2 - y1)^2 + (x2 - x1)^2);

end


% Compute the relative angle of angle2 wrt angle1
function ret = computeRelativeAngle(angle1, angle2)

ret = angle2 - angle1;
% set return angle such that -pi < ret <= pi
ret = abs_lt_pi(ret);

end


% Compute the global angle of p2 wrt p1
function ret = computeGlobalAngle(p1, p2)

ret = atan2(p2(2) - p1(2), p2(1) - p1(1));
% set return angle such that -pi < ret <= pi
ret = abs_lt_pi(ret);

end


% "Abs(angle) less than pi"
% set angle such that -pi < angle <= pi
function ret = abs_lt_pi(angle)

while(angle > pi)
    angle = angle - 2 * pi;
end
while(angle <= -pi)
    angle = angle + 2 * pi;
end
% set return value
ret = angle;

end

== matlab function RL_Model_dyn/Output Conversion/MATLAB Function ==
  data: u input; y output
function y = fcn(u)
coder.extrinsic('evalin', 'assignin');
assignin('base', 'ang_velocity', u);
y = u;

== matlab function RL_Model_dyn/NN_trainer/simul ==
  data: u input; y output
function y = fcn(u)


coder.extrinsic('evalin', 'assignin');

started = false;
is_sim = false;

started = evalin('base', 'started');
is_sim = evalin('base', 'is_sim');

%load error.mat
%load error_retrained1.mat
%persistent started;
%if isempty(started)
%    started = 1;
%end

second_if_flag = true;
second_if_flag = evalin('base', 'second_if_flag');

if (u && is_sim && (started == false))
    error_data = evalin('base', 'error_data');
    temp_error_for_nn_emul = evalin('base', 'temp_error_for_nn_emul');
    
    error_data = abs(error_data);
    error_mean = mean(error_data);
    error_max = max(error_data);
    error_for_nn_emul = temp_error_for_nn_emul;    
                         
    assignin('base', 'error_for_nn_emul', error_for_nn_emul);
    assignin('base', 'error_mean', error_mean);
    assignin('base', 'error_max', error_max);
    
    
elseif (u && is_sim && started && second_if_flag)
    
    error_data = evalin('base', 'error_data');
    error_mean = evalin('base', 'error_mean');
    error_max = evalin('base', 'error_max');
    error_for_nn_emul = evalin('base', 'error_for_nn_emul');
    temp_error_for_nn_emul = evalin('base', 'temp_error_for_nn_emul');
    
    error_data = abs(error_data);
    error_mean = [error_mean;
                  mean(error_data)]
    error_max = [error_max;
                 max(error_data)]
             
    
    error_for_nn_emul = [error_for_nn_emul;
                              temp_error_for_nn_emul];
    assignin('base', 'error_for_nn_emul', error_for_nn_emul);
        
    assignin('base', 'error_mean', error_mean);
    assignin('base', 'error_max', error_max);
    
    second_if_flag = false;
    assignin('base', 'second_if_flag', second_if_flag);

end




y = u;

== matlab function RL_Model_dyn/NN_trainer/Plotter ==
  data: u input; y output
function y = fcn(u)

coder.extrinsic('plotpath', 'evalin', 'assignin');

persistent plotFlag;
if isempty(plotFlag)
    plotFlag = true;
end

if (u && plotFlag)

    % import variables from workspace
    graph_vars = evalin('base', 'graph_vars');
    temp_position_data = evalin('base', 'temp_position_data');
    temp_error_data = evalin('base', 'temp_error_data');
    
    position_data = temp_position_data;
    error_data = temp_error_data;
    
    assignin('base', 'position_data', position_data);
    assignin('base', 'error_data', error_data);
    
    plotpath(graph_vars, position_data)
    plotFlag = false;
    
end

y = u;
